simulink model "PID_left_wheels2015a"  (Simulink 8.5)
settings: Solver=ode4  StartTime=0.0  StopTime=50  FixedStep=0.01  RelTol=1e-6
settings Model: Creator=Rafael  LastModifiedBy=root
settings DataIOCC: SignalLoggingSaveFormat=Dataset
settings OptimizationCC: ExpressionDepthLimit=128
settings DebuggingCC: UnderspecifiedInitializationDetection=Simplified  MergeDetectMultiDrivingBlocksExec=error  FcnCallInpInsideContextMsg=EnableAllAsError  StateNameClashWarn=none
settings GRTTargetCC: CombineOutputUpdateFcns=on  GRTInterface=off

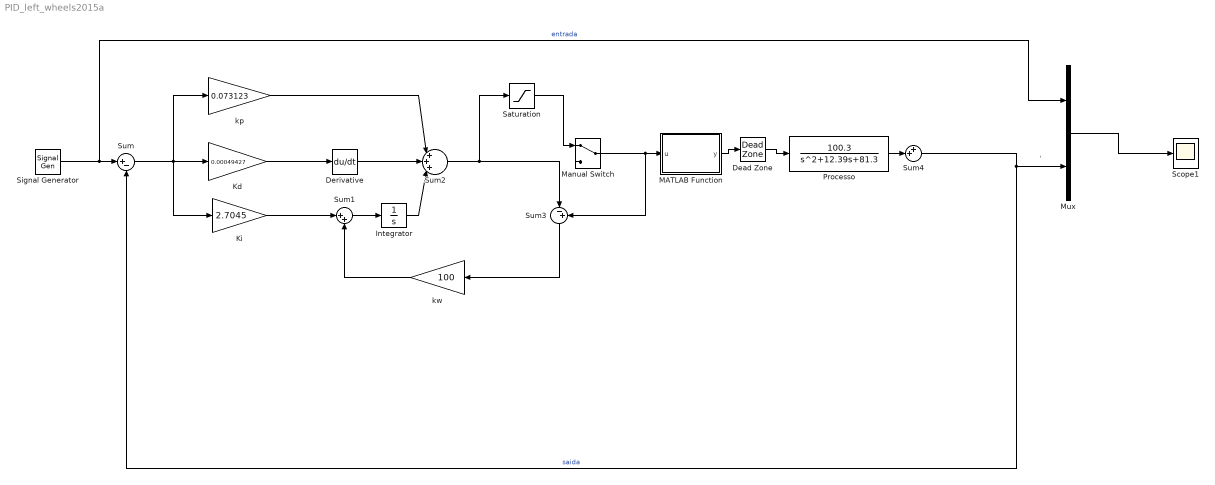
== system PID_left_wheels2015a ==
  note: '
  Dead Zone : DeadZone  LowerValue=-1  UpperValue=1  SaturateOnIntegerOverflow=on
  Derivative : Derivative
  Integrator : Integrator
  Kd : Gain  Gain=0.00049427
  Ki : Gain  Gain=2.7045
  MATLAB Function : MATLAB Function  TreatAsAtomicUnit=on
      settings: PermitHierarchicalResolution=ParametersOnly
  Manual Switch : ManualSwitch
  Mux : Mux  Inputs=2
  Processo : TransferFcn  Numerator=[100.3]  Denominator=[1 12.39 81.3]
  Saturation : Saturate  UpperLimit=6  LowerLimit=-6
  Scope1 : Scope
      settings: TimeRange=auto  LimitDataPoints=on  MaxDataPoints=5000  SaveToWorkspace=off  SaveName=ScopeData  YMin=-8.75  YMax=8.75  SampleTime=-1  DataFormat=Array
  Signal Generator : SignalGenerator  WaveForm=square  Amplitude=7  Frequency=0.08
  Sum : Sum  Inputs=|+-
  Sum1 : Sum  Inputs=|++
  Sum2 : Sum  Inputs=|+++|
  Sum3 : Sum  Inputs=|-+
  Sum4 : Sum  Inputs=++|
  kp : Gain  Gain=0.073123
  "kw " : Gain  Gain=100
  wires:
  Dead Zone/1 -> Processo/1
  Sum/1 -> kp/1, Kd/1, Ki/1
  kp/1 -> Sum2/1
  Derivative/1 -> Sum2/2
  Sum1/1 -> Integrator/1
  Integrator/1 -> Sum2/3
  Manual Switch/1 -> MATLAB Function/1(u), Sum3/2
  Saturation/1 -> Manual Switch/1
  Sum4/1 -> Sum/2, Mux/2  "saida"
  Processo/1 -> Sum4/2
  Signal Generator/1 -> Mux/1, Sum/1  "entrada"
  Kd/1 -> Derivative/1
  MATLAB Function/1(y) -> Dead Zone/1
  Ki/1 -> Sum1/1
  "kw "/1 -> Sum1/2
  Mux/1 -> Scope1/1
  Sum3/1 -> "kw "/1
  Sum2/1 -> Sum3/1, Saturation/1

== matlab function MATLAB Function ==
  data: u input double; y output double
function y = inverte(u)
if (u > 0)
    u = u + 1;
end 
if (u <= 0)
    u = u - 1;
end 
y = u;
